simulink model "Example_S_Function"  (R2013a)
settings: Solver=ode45  StartTime=0.0  StopTime=7.5  RelTol=1e-3
settings Model: Creator=awohlfei  LastModifiedBy=awohlfei

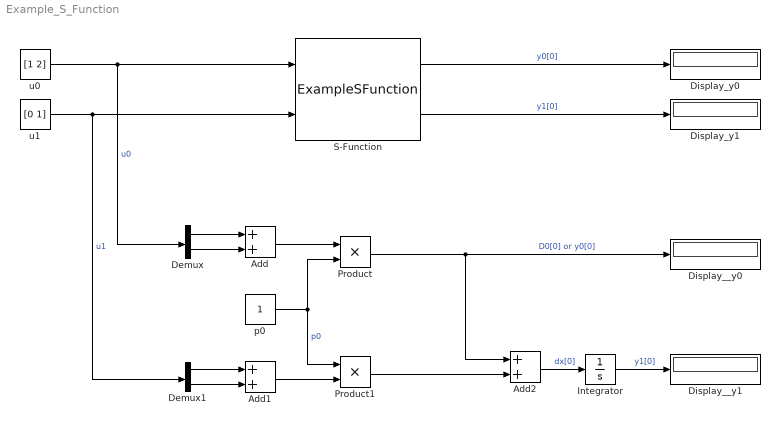
== system Example_S_Function ==
  Add : Sum
  Add1 : Sum
  Add2 : Sum
  Demux : Demux  Outputs=2
  Demux1 : Demux  Outputs=2
  Display__y0 : Display
  Display__y1 : Display
  Display_y0 : Display
  Display_y1 : Display
  Integrator : Integrator
  Product : Product
  Product1 : Product
  S-Function : S-Function  FunctionName=ExampleSFunction  Parameters=1  EnableBusSupport=off
  p0 : Constant
  u0 : Constant  Value=[1 2]
  u1 : Constant  Value=[0 1]
  wires:
  u0/1 -> Demux/1, S-Function/1  "u0"
  Demux/1 -> Add/1
  Demux/2 -> Add/2
  u1/1 -> Demux1/1, S-Function/2  "u1"
  Demux1/1 -> Add1/1
  Demux1/2 -> Add1/2
  Add/1 -> Product/1
  p0/1 -> Product1/1, Product/2  "p0"
  Add1/1 -> Product1/2
  Product1/1 -> Add2/2
  S-Function/1 -> Display_y0/1  "y0[0]"
  S-Function/2 -> Display_y1/1  "y1[0]"
  Product/1 -> Add2/1, Display__y0/1  "D0[0] or y0[0]"
  Integrator/1 -> Display__y1/1  "y1[0]"
  Add2/1 -> Integrator/1  "dx[0]"
